simulink model "ROSFeedBackExample"  (R2019b)
settings: Solver=FixedStepDiscrete  StartTime=0.0  StopTime=Inf  FixedStep=0.02  RelTol=1e-3  EnableMultiTasking=on
values from neighbouring files (symbols this model uses):
  m = size(BW, 1)    [ClusterClean.m]    (also in ClusterFuck.m; dotDetection.m)
  X = (round((Ball{1,2}-571)*pixel2mm,2))    [ClusterClean.m]    (also in ClusterFuck.m = (round((Ball{1,2}-CueX)*pixel2mm+30-6.275,2)); PossibleShots.m = (round((balls{1,2})*pixel2mm,2)-6.71); dotDetection.m = rgb2lab(img))
  Y = (round((Ball{1,3}-41)*pixel2mm,2))    [ClusterClean.m]    (also in ClusterFuck.m = (round((Ball{1,3}-CueY)*pixel2mm+30,2)); PossibleShots.m = (round((balls{1,3})*pixel2mm,2)-6.71))
  Z = 80    [ClusterClean.m]    (also in ClusterFuck.m = 90; PossibleShots.m = 90)
undefined symbols (not defined in the file or in its folder): Angular, awayFromGoalThresh, Linear, loadingStation, logicalMap, objectPos, p, q0, refPos, tDuration, tStart, unloadingStations
libraries: sm_lib x153, nesl_utility x33, robotlib x7, robotmaniplib x5, simulink x3, robotalgslib x1
(part 4 of 4)

== system ROSFeedBackExample/Perform Safe Trajectory Tracking Control Using Robotics Manipulator Blocks/Simscape Model with Simple Contact Mechanics/right_torso_itb1 ==
  Inertia : sm_lib/Body Elements/Spherical Solid  GraphicAmbientColor=[0.15 0.15 0.15 1.0]  BasedOnType=Density  CenterOfMass=[0, 0, 0]  CenterOfMassUnits=m  GraphicDiffuseColor=[0.5 0.5 0.5]  Density=1000  DensityUnits=kg/m^3  DoExposeReferenceFrame=on  GraphicEmissiveColor=[0.0 0.0 0.0 1.0]  ExportEntireGeometry=off  SerializedExposedGeometries=<ExposedGeometries/>  SerializedFrames=<Frames/>  MarkerShape=Sphere  MarkerSize=10  GraphicType=None  InertiaType=Custom  Mass=0.0001  MassUnits=kg  MomentsOfInertia=[1e-08, 1e-08, 1e-08]  MomentsOfInertiaUnits=kg*m^2  GraphicOpacity=1.0  ProductsOfInertia=[0, 0, 0]  ProductsOfInertiaUnits=kg*m^2  GraphicShininess=75  GraphicSpecularColor=[0.5 0.5 0.5 1.0]  SphereRadius=1  SphereRadiusUnits=m  GraphicVisPropType=SimpleVisualProperties
      settings: SourceProductName=Simscape Multibody
  InertiaOriginTransform : sm_lib/Frames and Transforms/Rigid Transform  TranslationMethod=Cartesian  TranslationStandardOffset=0  TranslationLengthUnit=m  TranslationStandardAxis=+Z  TranslationCartesianOffset=[0, 0, 0]  TranslationROffset=0  TranslationROffsetUnits=m  TranslationZOffset=0  TranslationZOffsetUnits=m  TranslationThetaOffset=0  TranslationThetaOffsetUnits=deg  RotationMethod=RotationSequence  RotationAngleUnits=deg  RotationStandardAxis=+Z  RotationAngle=0.0  RotationArbitraryAxis=[0 0 1]  FollAlignAxisA=+X  BaseAlignAxisA=+Y  FollAlignAxisB=+Y  BaseAlignAxisB=+Z  RotationSequenceAxes=BaseAxes  RotationSequence=XYZ  RotationSequenceAngles=[0, 0, 0]  RotationSequenceAnglesUnits=rad  RotationMatrix=[1 0 0; 0 1 0; 0 0 1]
  ReferenceFrame : sm_lib/Frames and Transforms/Reference Frame
  F : PMIOPort  Side=Left
  connections:
  Inertia/RConn1 -- InertiaOriginTransform/RConn1
  ReferenceFrame/RConn1 -- InertiaOriginTransform/LConn1 -- F/RConn1

== system ROSFeedBackExample/Perform Safe Trajectory Tracking Control Using Robotics Manipulator Blocks/Simscape Model with Simple Contact Mechanics/right_wrist1 ==
  ReferenceFrame : sm_lib/Frames and Transforms/Reference Frame
  F : PMIOPort  Side=Left
  connections:
  ReferenceFrame/RConn1 -- F/RConn1

== system ROSFeedBackExample/Perform Safe Trajectory Tracking Control Using Robotics Manipulator Blocks/Simscape Model with Simple Contact Mechanics/screen ==
  Inertia : sm_lib/Body Elements/Spherical Solid  GraphicAmbientColor=[0.15 0.15 0.15 1.0]  BasedOnType=Density  CenterOfMass=[0, 0, 0]  CenterOfMassUnits=m  GraphicDiffuseColor=[0.5 0.5 0.5]  Density=1000  DensityUnits=kg/m^3  DoExposeReferenceFrame=on  GraphicEmissiveColor=[0.0 0.0 0.0 1.0]  ExportEntireGeometry=off  SerializedExposedGeometries=<ExposedGeometries/>  SerializedFrames=<Frames/>  MarkerShape=Sphere  MarkerSize=10  GraphicType=None  InertiaType=Custom  Mass=0.0001  MassUnits=kg  MomentsOfInertia=[1e-08, 1e-08, 1e-08]  MomentsOfInertiaUnits=kg*m^2  GraphicOpacity=1.0  ProductsOfInertia=[0, 0, 0]  ProductsOfInertiaUnits=kg*m^2  GraphicShininess=75  GraphicSpecularColor=[0.5 0.5 0.5 1.0]  SphereRadius=1  SphereRadiusUnits=m  GraphicVisPropType=SimpleVisualProperties
      settings: SourceProductName=Simscape Multibody
  InertiaOriginTransform : sm_lib/Frames and Transforms/Rigid Transform  TranslationMethod=Cartesian  TranslationStandardOffset=0  TranslationLengthUnit=m  TranslationStandardAxis=+Z  TranslationCartesianOffset=[0, 0, 0]  TranslationROffset=0  TranslationROffsetUnits=m  TranslationZOffset=0  TranslationZOffsetUnits=m  TranslationThetaOffset=0  TranslationThetaOffsetUnits=deg  RotationMethod=RotationSequence  RotationAngleUnits=deg  RotationStandardAxis=+Z  RotationAngle=0.0  RotationArbitraryAxis=[0 0 1]  FollAlignAxisA=+X  BaseAlignAxisA=+Y  FollAlignAxisB=+Y  BaseAlignAxisB=+Z  RotationSequenceAxes=BaseAxes  RotationSequence=XYZ  RotationSequenceAngles=[0, 0, 0]  RotationSequenceAnglesUnits=rad  RotationMatrix=[1 0 0; 0 1 0; 0 0 1]
  ReferenceFrame : sm_lib/Frames and Transforms/Reference Frame
  Visual : sm_lib/Body Elements/Brick Solid  GraphicAmbientColor=[0.15 0.15 0.15 1.0]  BasedOnType=Density  BrickDimensions=[0.24, 0.14, 0.002]  BrickDimensionUnits=m  CenterOfMass=[0, 0, 0]  CenterOfMassUnits=m  GraphicDiffuseColor=[0.2, 0.2, 0.2]  Density=1000  DensityUnits=kg/m^3  DoExposeReferenceFrame=on  GraphicEmissiveColor=[0.0 0.0 0.0 1.0]  ExportEntireGeometry=off  SerializedFrames=<Frames/>  MarkerShape=Sphere  MarkerSize=10  GraphicType=FromGeometry  InertiaType=Custom  Mass=0  MassUnits=kg  MomentsOfInertia=[0, 0, 0]  MomentsOfInertiaUnits=kg*m^2  GraphicOpacity=1  ProductsOfInertia=[0, 0, 0]  ProductsOfInertiaUnits=kg*m^2  GraphicShininess=75  GraphicSpecularColor=[0.5 0.5 0.5 1.0]  GraphicVisPropType=SimpleVisualProperties
  VisualOriginTransform : sm_lib/Frames and Transforms/Rigid Transform  TranslationMethod=Cartesian  TranslationStandardOffset=0  TranslationLengthUnit=m  TranslationStandardAxis=+Z  TranslationCartesianOffset=[0, 0, 0]  TranslationROffset=0  TranslationROffsetUnits=m  TranslationZOffset=0  TranslationZOffsetUnits=m  TranslationThetaOffset=0  TranslationThetaOffsetUnits=deg  RotationMethod=RotationSequence  RotationAngleUnits=deg  RotationStandardAxis=+Z  RotationAngle=0.0  RotationArbitraryAxis=[0 0 1]  FollAlignAxisA=+X  BaseAlignAxisA=+Y  FollAlignAxisB=+Y  BaseAlignAxisB=+Z  RotationSequenceAxes=BaseAxes  RotationSequence=XYZ  RotationSequenceAngles=[0, 0, 0]  RotationSequenceAnglesUnits=rad  RotationMatrix=[1 0 0; 0 1 0; 0 0 1]
  F : PMIOPort  Side=Left
  connections:
  Inertia/RConn1 -- InertiaOriginTransform/RConn1
  ReferenceFrame/RConn1 -- InertiaOriginTransform/LConn1 -- VisualOriginTransform/LConn1 -- F/RConn1
  Visual/RConn1 -- VisualOriginTransform/RConn1

== system ROSFeedBackExample/Perform Safe Trajectory Tracking Control Using Robotics Manipulator Blocks/Simscape Model with Simple Contact Mechanics/torso ==
  Inertia : sm_lib/Body Elements/Spherical Solid  GraphicAmbientColor=[0.15 0.15 0.15 1.0]  BasedOnType=Density  CenterOfMass=[0, 0, 0]  CenterOfMassUnits=m  GraphicDiffuseColor=[0.5 0.5 0.5]  Density=1000  DensityUnits=kg/m^3  DoExposeReferenceFrame=on  GraphicEmissiveColor=[0.0 0.0 0.0 1.0]  ExportEntireGeometry=off  SerializedExposedGeometries=<ExposedGeometries/>  SerializedFrames=<Frames/>  MarkerShape=Sphere  MarkerSize=10  GraphicType=None  InertiaType=Custom  Mass=0.0001  MassUnits=kg  MomentsOfInertia=[1e-08, 1e-08, 1e-08]  MomentsOfInertiaUnits=kg*m^2  GraphicOpacity=1.0  ProductsOfInertia=[0, 0, 0]  ProductsOfInertiaUnits=kg*m^2  GraphicShininess=75  GraphicSpecularColor=[0.5 0.5 0.5 1.0]  SphereRadius=1  SphereRadiusUnits=m  GraphicVisPropType=SimpleVisualProperties
      settings: SourceProductName=Simscape Multibody
  InertiaOriginTransform : sm_lib/Frames and Transforms/Rigid Transform  TranslationMethod=Cartesian  TranslationStandardOffset=0  TranslationLengthUnit=m  TranslationStandardAxis=+Z  TranslationCartesianOffset=[0, 0, 0]  TranslationROffset=0  TranslationROffsetUnits=m  TranslationZOffset=0  TranslationZOffsetUnits=m  TranslationThetaOffset=0  TranslationThetaOffsetUnits=deg  RotationMethod=RotationSequence  RotationAngleUnits=deg  RotationStandardAxis=+Z  RotationAngle=0.0  RotationArbitraryAxis=[0 0 1]  FollAlignAxisA=+X  BaseAlignAxisA=+Y  FollAlignAxisB=+Y  BaseAlignAxisB=+Z  RotationSequenceAxes=BaseAxes  RotationSequence=XYZ  RotationSequenceAngles=[0, 0, 0]  RotationSequenceAnglesUnits=rad  RotationMatrix=[1 0 0; 0 1 0; 0 0 1]
  ReferenceFrame : sm_lib/Frames and Transforms/Reference Frame
  Visual : sm_lib/Body Elements/Brick Solid  GraphicAmbientColor=[0.15 0.15 0.15 1.0]  BasedOnType=Density  BrickDimensions=[0.001, 0.001, 0.001]  BrickDimensionUnits=m  CenterOfMass=[0, 0, 0]  CenterOfMassUnits=m  GraphicDiffuseColor=[0.2, 0.2, 0.2]  Density=1000  DensityUnits=kg/m^3  DoExposeReferenceFrame=on  GraphicEmissiveColor=[0.0 0.0 0.0 1.0]  ExportEntireGeometry=off  SerializedFrames=<Frames/>  MarkerShape=Sphere  MarkerSize=10  GraphicType=FromGeometry  InertiaType=Custom  Mass=0  MassUnits=kg  MomentsOfInertia=[0, 0, 0]  MomentsOfInertiaUnits=kg*m^2  GraphicOpacity=1  ProductsOfInertia=[0, 0, 0]  ProductsOfInertiaUnits=kg*m^2  GraphicShininess=75  GraphicSpecularColor=[0.5 0.5 0.5 1.0]  GraphicVisPropType=SimpleVisualProperties
  VisualOriginTransform : sm_lib/Frames and Transforms/Rigid Transform  TranslationMethod=Cartesian  TranslationStandardOffset=0  TranslationLengthUnit=m  TranslationStandardAxis=+Z  TranslationCartesianOffset=[0, 0, 0]  TranslationROffset=0  TranslationROffsetUnits=m  TranslationZOffset=0  TranslationZOffsetUnits=m  TranslationThetaOffset=0  TranslationThetaOffsetUnits=deg  RotationMethod=RotationSequence  RotationAngleUnits=deg  RotationStandardAxis=+Z  RotationAngle=0.0  RotationArbitraryAxis=[0 0 1]  FollAlignAxisA=+X  BaseAlignAxisA=+Y  FollAlignAxisB=+Y  BaseAlignAxisB=+Z  RotationSequenceAxes=BaseAxes  RotationSequence=XYZ  RotationSequenceAngles=[0, 0, 0]  RotationSequenceAnglesUnits=rad  RotationMatrix=[1 0 0; 0 1 0; 0 0 1]
  F : PMIOPort  Side=Left
  connections:
  Inertia/RConn1 -- InertiaOriginTransform/RConn1
  ReferenceFrame/RConn1 -- InertiaOriginTransform/LConn1 -- VisualOriginTransform/LConn1 -- F/RConn1
  Visual/RConn1 -- VisualOriginTransform/RConn1

== system ROSFeedBackExample/Perform Safe Trajectory Tracking Control Using Robotics Manipulator Blocks/Trajectory Scaling and Desired Motion/Clock with Switch ==
  t_In : Inport
  Constant1 : Constant  Value=tStart
  If : If  NumInputs=2  IfExpression=u1 >u2  ShowElse=off
  If Action Subsystem : Subsystem  TreatAsAtomicUnit=on
  Scope : Scope
  t_Out : Outport  VectorParamsAs1DForOutWhenUnconnected=off
  wires:
  t_In/1 -> If/1, If Action Subsystem/1(In1)
  If Action Subsystem/1(Out1) -> t_Out/1, Scope/1
  If/1 -> If Action Subsystem/Action
  Constant1/1 -> If Action Subsystem/2(In2), If/2

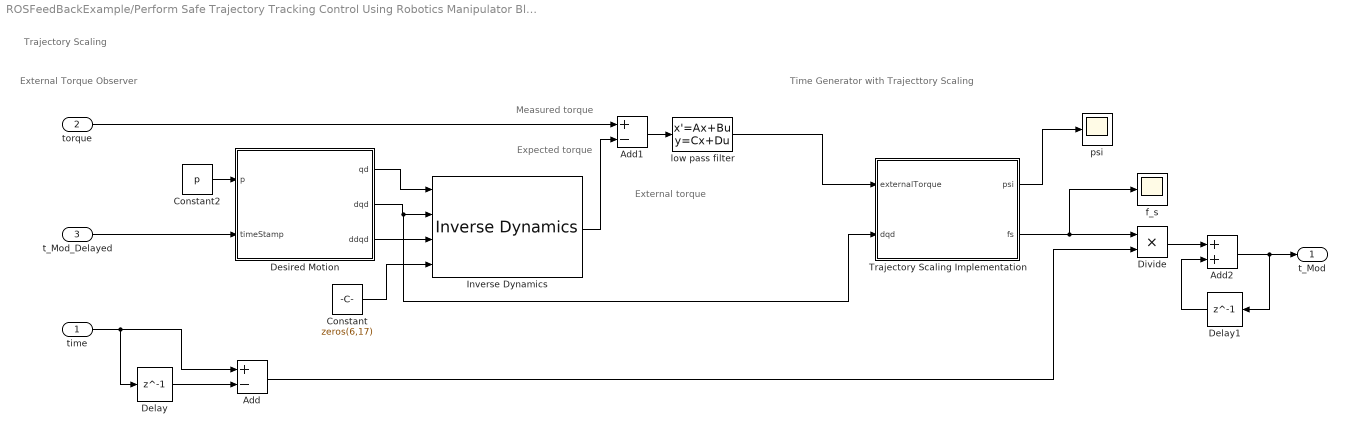
== system ROSFeedBackExample/Perform Safe Trajectory Tracking Control Using Robotics Manipulator Blocks/Trajectory Scaling and Desired Motion/Trajectory Scaling ==
  note: External torque
  note: External Torque Observer
  note: Time Generator with Trajecttory Scaling
  note: Trajectory Scaling
  note: Measured torque
  note: Expected torque
  time : Inport
  torque : Inport  Port=2
  "t_Mod_Delayed " : Inport  Port=3
  Add : Sum  Inputs=+-
  Add1 : Sum  Inputs=+-
  Add2 : Sum
  Constant : Constant  Value=zeros(6,17)
  Constant2 : Constant  Value=p
  Delay : Delay  DelayLength=1
  Delay1 : Delay  DelayLength=1
  Desired Motion : MATLAB Function  TreatAsAtomicUnit=on
  Divide : Product  Inputs=**
  Inverse Dynamics : robotmaniplib/Inverse Dynamics  RigidBodyTree=sawyer  SimulateUsing=Interpreted execution
      settings: SourceProductName=Robotics System Toolbox  SourceProductBaseCode=RO
  Trajectory Scaling Implementation : MATLAB Function  TreatAsAtomicUnit=on
  f_s : Scope
  low pass filter : StateSpace  A=-50*eye(7)  B=50*eye(7)  C=eye(7)  D=zeros(7,7)  InitialCondition=zeros(7,1)
  psi : Scope
  t_Mod : Outport  VectorParamsAs1DForOutWhenUnconnected=off
  wires:
  Trajectory Scaling Implementation/1(psi) -> psi/1
  Trajectory Scaling Implementation/2(fs) -> f_s/1, Divide/1
  Delay/1 -> Add/2
  Divide/1 -> Add2/1
  time/1 -> Delay/1, Add/1
  Add2/1 -> Delay1/1, t_Mod/1
  Constant2/1 -> Desired Motion/1(p)
  "t_Mod_Delayed "/1 -> Desired Motion/2(timeStamp)
  Desired Motion/1(qd) -> Inverse Dynamics/1
  Desired Motion/2(dqd) -> Trajectory Scaling Implementation/2(dqd), Inverse Dynamics/2
  Desired Motion/3(ddqd) -> Inverse Dynamics/3
  torque/1 -> Add1/1
  Inverse Dynamics/1 -> Add1/2
  Constant/1 -> Inverse Dynamics/4
  Add/1 -> Divide/2
  Add1/1 -> low pass filter/1
  low pass filter/1 -> Trajectory Scaling Implementation/1(externalTorque)
  Delay1/1 -> Add2/2

== system ROSFeedBackExample/Perform Safe Trajectory Tracking Control Using Robotics Manipulator Blocks/Simscape Model with Simple Contact Mechanics/Contact Force and Planar Object Motion and Visualization/Planar Object ==
  Inertia : sm_lib/Body Elements/Brick Solid  GraphicAmbientColor=[0.15 0.15 0.15 1.0]  BasedOnType=Density  BrickDimensions=[0.1 1 1]  BrickDimensionUnits=m  CenterOfMass=[0, 0, 0]  CenterOfMassUnits=m  GraphicDiffuseColor=[0.5 0.5 0.5]  Density=1000  DensityUnits=kg/m^3  DoExposeReferenceFrame=on  GraphicEmissiveColor=[0.0 0.0 0.0 1.0]  ExportEntireGeometry=off  SerializedFrames=<Frames/>  MarkerShape=Sphere  MarkerSize=10  GraphicType=FromGeometry  InertiaType=Custom  Mass=1e8  MassUnits=kg  MomentsOfInertia=[1e-08, 1e-08, 1e-08]  MomentsOfInertiaUnits=kg*m^2  GraphicOpacity=1  ProductsOfInertia=[1e-08, 1e-08, 1e-08]  ProductsOfInertiaUnits=kg*m^2  GraphicShininess=75  GraphicSpecularColor=[0.5 0.5 0.5 1.0]  GraphicVisPropType=SimpleVisualProperties
  InertiaOriginTransform : sm_lib/Frames and Transforms/Rigid Transform  TranslationMethod=Cartesian  TranslationStandardOffset=0  TranslationLengthUnit=m  TranslationStandardAxis=+Z  TranslationCartesianOffset=[1e-08, 1e-08, 1e-08]  TranslationROffset=0  TranslationROffsetUnits=m  TranslationZOffset=0  TranslationZOffsetUnits=m  TranslationThetaOffset=0  TranslationThetaOffsetUnits=deg  RotationMethod=RotationSequence  RotationAngleUnits=deg  RotationStandardAxis=+Z  RotationAngle=0.0  RotationArbitraryAxis=[0 0 1]  FollAlignAxisA=+X  BaseAlignAxisA=+Y  FollAlignAxisB=+Y  BaseAlignAxisB=+Z  RotationSequenceAxes=BaseAxes  RotationSequence=XYZ  RotationSequenceAngles=[0, 0, 0]  RotationSequenceAnglesUnits=rad  RotationMatrix=[1 0 0; 0 1 0; 0 0 1]
  ReferenceFrame : sm_lib/Frames and Transforms/Reference Frame
  F : PMIOPort  Side=Left
  connections:
  Inertia/RConn1 -- InertiaOriginTransform/RConn1
  ReferenceFrame/RConn1 -- InertiaOriginTransform/LConn1 -- F/RConn1

== system ROSFeedBackExample/Perform Safe Trajectory Tracking Control Using Robotics Manipulator Blocks/Trajectory Scaling and Desired Motion/Clock with Switch/If Action Subsystem ==
  In1 : Inport
  In2 : Inport  Port=2
  Action Port : ActionPort
  Add : Sum  Inputs=+-
  Out1 : Outport  VectorParamsAs1DForOutWhenUnconnected=off
  wires:
  In1/1 -> Add/1
  Add/1 -> Out1/1
  In2/1 -> Add/2

== matlab function ROSFeedBackExample/Get cord and adjust Example/Conversion ==
  data: yaw output; x input; y input; z input; w input
function yaw  = quat2eul(x,y,z,w)
%#codegen

% Convert the quaternion to a yaw angle (zyx euler angle)
eul = quat2eul([w,x,y,z]);
yaw = eul(1);

end

== matlab function ROSFeedBackExample/Point cloud Example/MATLAB Function ==
  data: comXYZ output; xyzPoints input
function comXYZ = pointCloudCOM(xyzPoints)
% Compute the center of mass of a point cloud based on the input NxMx3
% matrix.

% Turn matrix into vectors.
xPoints = reshape(xyzPoints(:,:,1),numel(xyzPoints(:,:,1)),1);
yPoints = reshape(xyzPoints(:,:,2),numel(xyzPoints(:,:,2)),1);
zPoints = reshape(xyzPoints(:,:,3),numel(xyzPoints(:,:,3)),1);

% Calculate the mean for each set of coordiantes.
xMean = mean(xPoints,'omitnan');
yMean = mean(yPoints,'omitnan');
zMean = mean(zPoints,'omitnan');

comXYZ = [xMean,yMean,zMean];

end

== matlab function ROSFeedBackExample/Subsystem/Planner ==
  settings: updateMethod=DISCRETE
  data: startPos input size=[1 2]; endPos input size=[1 2]; waypoints output size=[100 2]; mapMatrix input
function waypoints = planning(startPos, endPos, mapMatrix)

persistent waypointsInternal
persistent prevStartPos
persistent prevEndPos

% Set constant parameters
maxNumNodes = 100;

% Initialize persistent variables that are used downstream
if isempty(prevStartPos)
    prevStartPos = startPos;
end

if isempty(prevEndPos)
    prevEndPos = endPos;
end

isNewPath = (~isequal(prevStartPos, startPos) || ~isequal(prevEndPos, endPos));

if isempty(waypointsInternal) || isNewPath
    % Two conditions in which waypoints must be set: they are not yet
    % initialized, or they are initialized, but the current start and end
    % do not match those used to generate the previous set of waypoints
    [waypointsInternal] = planPath(mapMatrix, maxNumNodes, startPos, endPos);
end

% Update the outputs
waypoints = waypointsInternal;

% Update the persistent variables that indicate previous state
prevStartPos = startPos;
prevEndPos = endPos;

%% Helper Function



end

function wayPoints = planPath(mapMatrix, maxNodes, startPos, endPos)
    
    % Create a probabilistic roadmap
    map = binaryOccupancyMap(mapMatrix);
    prm = mobileRobotPRM(map, maxNodes);
    
    % Find a path between two points
    xy = findpath(prm, startPos, endPos);
    wayPoints = repmat(endPos, maxNodes, 1);
    
    % Number of nodes that are actually used
    numNodes = length(xy);
    wayPoints(1:numNodes,:) = xy;    

end

== stateflow chart ROSFeedBackExample/Subsystem/Scheduler ==
  settings: sampleTime=0.1
  state GoToUnloadingStation
    entry:
    robotGoal = unloadingStations(package, :)';
    robotStart = currentPose(1:2)';
  state GoToLoadingStation
    entry:
    robotGoal = loadingStation';
    robotStart = currentPose(1:2)';
  state StationHalt
    entry, during:
  (default) -> (junction 65) : {robotStart = startPose;
      | hasPackage = 0;
      | }
  (junction 65) -> GoToLoadingStation
  GoToLoadingStation -> StationHalt [order 1] : [hasPackage && package]
  StationHalt -> GoToUnloadingStation [order 1] : [planningState == RobotState.AtLoadingStn && ...
      | after(stopDelay, tick)]
  StationHalt -> GoToLoadingStation [order 2] : [planningState == RobotState.AtUnloadingStn && ...
      | after(stopDelay, tick)]
  GoToUnloadingStation -> StationHalt : [~awayFromGoal]
      | {planningState = RobotState.AtUnloadingStn;
      | hasPackage = 0;}
  GoToLoadingStation -> (junction 72) [order 2] : [~awayFromGoal]{planningState = RobotState.AtLoadingStn;}
  (junction 72) -> (junction 102) : [receivedPackage]{hasPackage = 1;}
  data: hasPackage output; planningState output Enum: RobotState =RobotState.AtDock; loadingStation parameter; robotStart output size=[1, 2]; robotGoal output size=2; unloadingStations parameter; package input; receivedPackage input; currentPose input; startPose input size=[1 2]; awayFromGoal input; stopDelay local =0.5e3

== matlab function ROSFeedBackExample/Perform Safe Trajectory Tracking Control Using Robotics Manipulator Blocks/Trajectory Scaling and Desired Motion/Desired Motion ==
  data: p input; timeStamp input; qd output; dqd output; ddqd output
function [qd,dqd,ddqd] = trajEvaluation(p, timeStamp)
%trajEvaluation evaluates the desired motion
%   With the given polynomial coefficients of the generated trajectory and the 
%   time stamp, this function evaluates the desired position, velocity and
%   acceleration.

[qd,dqd,ddqd]= exampleHelperPolynomialTrajectoryEvaluation(p, timeStamp);

== matlab function ROSFeedBackExample/Perform Safe Trajectory Tracking Control Using Robotics Manipulator Blocks/Trajectory Scaling and Desired Motion/Trajectory Scaling/Desired Motion ==
  data: p input; timeStamp input; qd output; dqd output; ddqd output
function [qd,dqd,ddqd] = trajEvaluation(p, timeStamp)
%trajEvaluation evaluates the desired motion
%   With the given polynomial coefficients of the generated trajectory and the 
%   time stamp, this function evaluates the desired position, velocity and
%   acceleration.

[qd,dqd,ddqd]= exampleHelperPolynomialTrajectoryEvaluation(p, timeStamp);

== matlab function ROSFeedBackExample/Perform Safe Trajectory Tracking Control Using Robotics Manipulator Blocks/Simscape Model with Simple Contact Mechanics/Contact Force and Planar Object Motion and Visualization/Contact Model ==
  data: xPen input; vPen input; torque output; J input; force output; k input; d input
function [torque,force] = contactForce(xPen,vPen,J,k,d)
%contactForce calculates the reaction force and torque of the contact
%   The contact mechanism is modeled as a linear spring-damper system, and the
%   reaction force is calculated by the given penetration depth and
%   velocity. The torque applied on the robot due to the reaction force is
%   also calculated.

% Make sure the penetration depth is nonnegative  
if xPen<0
   xPen = 0;
end
% Make sure the penetration velocity is nonnegative  
if vPen<0
   vPen = 0;
end
% Calculate the reaction force based on a linear spring-damper model
force = -k*(xPen)-sign(xPen)*d*vPen;
fext = zeros(6,1);
fext(4) = force;
% Calculate the torque applied on the robot due to the reaction force
torque = J'*fext; 

end

== matlab function ROSFeedBackExample/Perform Safe Trajectory Tracking Control Using Robotics Manipulator Blocks/Trajectory Scaling and Desired Motion/Trajectory Scaling/Trajectory Scaling Implementation ==
  data: externalTorque input; dqd input; psi output; fs output
function [psi,fs] = func_fs(externalTorque, dqd)
%func_fs calculates the fs() based on the external torque and desired velocity
%   The scalar function fs(psi) is used for integrating the time stamp for 
%   trajectory scaling.
%
%   Reference:
%   [1] S. Haddadin, A. Albu-Schäffer, A. De Luca, and G. Hirzinger, 
%   “Collision detection and reaction: A contribution to safe physical 
%   human-robot interaction,” International Conference on Intelligent Robots 
%   and Systems, pp. 3356–3363, 2008.

% Calculate normalized dq
if norm(dqd)~=0
    dqd = dqd/norm(dqd);
else
    dqd = dqd*0;
end

% A constant to adjust the sensitivity of trajectory scaling
alpha = 0.1;

% Calculate psi based on dq and torque
psi = 1/alpha*(externalTorque'*dqd);
if psi<0
    psi = 0;
end

% Set Gamma as the dead zone for smooth transition between different range of psi
Gamma = 0.5;

% A constant gain for backward motion
k = 1;

% Calculate fs
fs = 1;
    if     0 <= psi && psi < 1
        % Adjust the robot motion speed for small interference 
        % (fs = 1 is the normal speed)
        fs = 1/2*(1+cos(pi*psi));
    elseif 1 <= psi && psi <= 1+Gamma
        % Make the robot stop for mild interference
        fs = 0;
    elseif 1+Gamma < psi && psi <= 2+Gamma
        % Make the robot move backward for large interference
        fs = k* 1/2*(1+cos((psi-1-Gamma)*pi))-k;
    elseif 2+Gamma < psi
        % Make the robot move backward with full speed determined by k
        fs = -k;
    end
end
